simulink model "work7_2_2"  (R2016a)
settings: Solver=VariableStepAuto  StartTime=0.0  StopTime=100  RelTol=1e-3
settings Model: Creator=AL  LastModifiedBy=AL

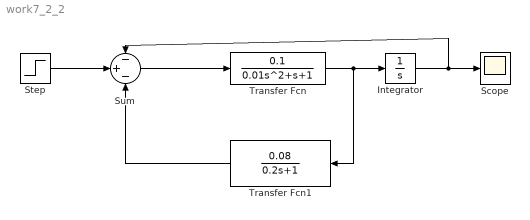
== system work7_2_2 ==
  Integrator : Integrator
  Scope : Scope
  Step : Step  SampleTime=0
  Sum : Sum  Inputs=-+-
  Transfer Fcn : TransferFcn  Numerator=[0.1]  Denominator=[0.01 1 1]
  Transfer Fcn1 : TransferFcn  Numerator=[0.08]  Denominator=[0.2 1]
  wires:
  Integrator/1 -> Scope/1, Sum/1
  Transfer Fcn/1 -> Transfer Fcn1/1, Integrator/1
  Sum/1 -> Transfer Fcn/1
  Transfer Fcn1/1 -> Sum/3
  Step/1 -> Sum/2
